simulink model "Test_Board"  (R2020a)
settings: Solver=FixedStepAuto  StartTime=0.0  StopTime=Inf  FixedStep=1e-3  RelTol=1e-3  EnableMultiTasking=on
undefined symbols (not defined in the file): D0, D1, D10, D11, D12, D13, D2, D3, D4, D5, D6, D7, D8, D9, PTA0, PTA1, PTA2, PTB23, PTB9, PTC16, PTC17, PTC2, PTC3, PTC4, PTD0, PTD1, PTD2, PTD3
libraries: frdmk64flib x18, dspstat3 x1
settings Model: ExtModeTrigDuration=5  Creator=Luis  LastModifiedBy=jordanbierbrier
settings OptimizationCC: EnhancedBackFolding=on  PassReuseOutputArgsAs=Individual arguments  ZeroExternalMemoryAtStartup=off  ZeroInternalMemoryAtStartup=off  MaxStackSize=64  OptimizeBlockOrder=speed  DifferentSizesBufferReuse=on  OptimizationCustomize=off  EfficientTunableParamExpr=on
settings DebuggingCC: ParameterTunabilityLossMsg=error
settings HardwareCC: ProdBitPerPointer=32  ProdBitPerSizeT=32  ProdBitPerPtrDiffT=32  ProdLargestAtomicInteger=Long  ProdLargestAtomicFloat=Double  ProdWordSize=32  ProdHWDeviceType=ARM Compatible->ARM Cortex
settings SFSimCC: MATLABDynamicMemAlloc=off
settings RTWCC: SystemTargetFile=ert.tlc  HardwareBoard=NXP FRDM-K64F  TemplateMakefile=ert_default_tmf  Toolchain=GNU Tools for ARM Embedded Processors
settings CodeAppCC: ForceParamTrailComments=on  IgnoreCustomStorageClasses=off  OperatorAnnotations=on  SimulinkDataObjDesc=on  SFDataObjDesc=on  InsertBlockDesc=on

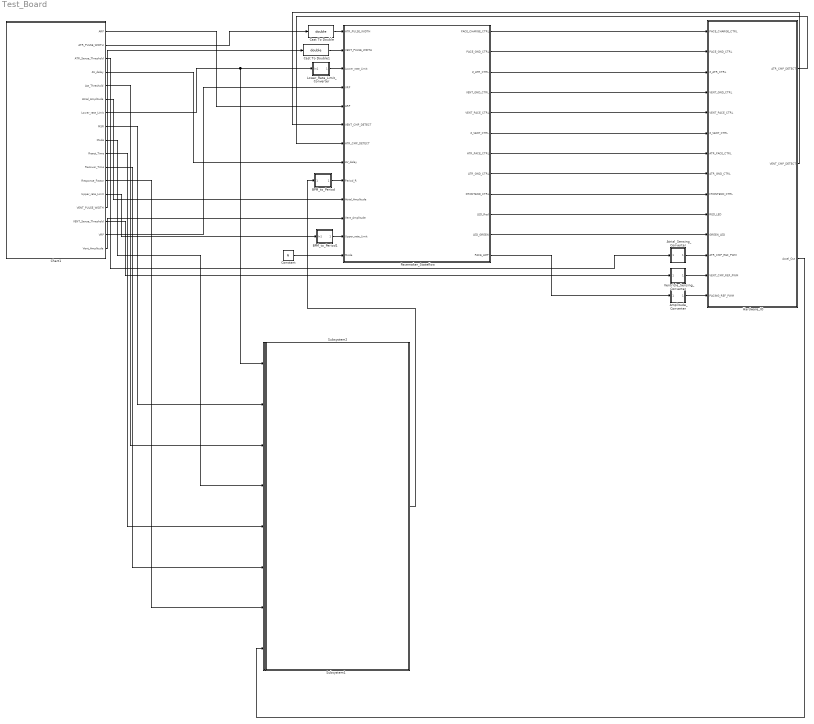
== system Test_Board ==
  Amplitude_Converter : Subsystem
  Atrial_Sensing_Converter : Subsystem
  BPM_to_Period : Subsystem
  BPM_to_Period1 : Subsystem
  Cast To Double : DataTypeConversion  OutDataTypeStr=double
  Cast To Double1 : DataTypeConversion  OutDataTypeStr=double
  Chart1 : Stateflow chart  TreatAsAtomicUnit=on
  Constant : Constant  Value=6  OutDataTypeStr=uint8
  Hardware_IO : Subsystem
  Lower_Rate_Limit_Converter : Subsystem
  "Pacemaker_Stateflow " : Stateflow chart  TreatAsAtomicUnit=on
      settings: PortSchema="{\"entries\":[{\"content\":{\"sides\":[{\"content\":{\"connectorIds\":[\"In1\",\"In4\",\"In2\",\"In5\",\"In6\",\"In7\",\"In8\",\"In9\",\"In10\",\"In11\",\"In12\",\"In13\",\"In3\"]},\"type\":\"ConnectorPlacement.EquallySpacedRectSide\",\"uuid\":\"f97b12ff-cb00-4386-a373-7143c3a8b48d\"},{\"content\":{\"connectorIds\":[\"Out1\",\"Out2\",\"Out3\",\"Out4\",\"Out5\",\"Out6\",\"Out7\",\"Out8\",\"Out9\",\"Out10\",\"Out11\",\"Out12\"],\"side\":\"RIGHT\"},\"type\":\"ConnectorPlacement.EquallySpacedRectSide\",\"uuid\":\"90163773-f9d1-46de-bd72-9589b8539202\"},{\"content\":{\"connectorIds\":[],\"side\":\"TOP\"},\"type\":\"ConnectorPlacement.EquallySpacedRectSide\",\"uuid\":\"f8a54119-a7c4-4071-8260-df405210e670\"},{\"content\":{\"connectorIds\":[],\"side\":\"BOTTOM\"},\"type\":\"ConnectorPlacement.EquallySpacedRectSide\",\"uuid\":\"70f9d800-d0b8-46e1-812e-9f4712f7acbd\"}]},\"type\":\"ConnectorPlacement.EquallySpacedConnector\",\"uuid\":\"47f7c40c-c42b-42f7-beed-99d299c6cdee\"}],\"packageUris\":[\"http://schema.mathworks.com/mf0/Connector/19700101\"],\"version\":\"1.0\"}"
  Subsystem1 : Subsystem
  Subsystem2 : Subsystem
  Ventricle_Sensing_Converter : Subsystem
  wires:
  Amplitude_Converter/1(Out1) -> Hardware_IO/14(PACING_REF_PWM)
  Chart1/13(Upper_rate_Limit) -> BPM_to_Period1/1(In1)
  Chart1/17(Vent_Amplitude) -> "Pacemaker_Stateflow "/12(Vent_Amplitude)
  Lower_Rate_Limit_Converter/1(Out1) -> "Pacemaker_Stateflow "/2(Lower_rate_Limit)
  Chart1/1(ARP) -> "Pacemaker_Stateflow "/6(ARP)
  BPM_to_Period1/1(Out1) -> "Pacemaker_Stateflow "/13(Upper_rate_Limit)
  "Pacemaker_Stateflow "/12(PACE_AMP) -> Amplitude_Converter/1(In1)
  Chart1/6(Atrial_Amplitude) -> "Pacemaker_Stateflow "/11(Atrial_Amplitude)
  Chart1/14(VENT_PULSE_WIDTH) -> Cast To Double1/1
  "Pacemaker_Stateflow "/2(PACE_GND_CTRL) -> Hardware_IO/2(PACE_GND_CTRL)
  "Pacemaker_Stateflow "/9(FRONTEND_CTRL) -> Hardware_IO/9(FRONTEND_CTRL)
  Chart1/10(React_Time) -> Subsystem1/5(Reaction)
  Chart1/12(Response_Factor) -> Subsystem1/7(Response_Factor)
  Cast To Double1/1 -> "Pacemaker_Stateflow "/4(VENT_PULSE_WIDTH)
  Chart1/3(ATR_Sense_Threshold) -> Atrial_Sensing_Converter/1(In1)
  "Pacemaker_Stateflow "/10(LED_Red) -> Hardware_IO/10(RED_LED)
  Chart1/4(AV_delay) -> "Pacemaker_Stateflow "/9(AV_delay)
  "Pacemaker_Stateflow "/7(ATR_PACE_CTRL) -> Hardware_IO/7(ATR_PACE_CTRL)
  "Pacemaker_Stateflow "/3(Z_ATR_CTRL) -> Hardware_IO/3(Z_ATR_CTRL)
  "Pacemaker_Stateflow "/8(ATR_GND_CTRL) -> Hardware_IO/8(ATR_GND_CTRL)
  "Pacemaker_Stateflow "/11(LED_GREEN) -> Hardware_IO/11(GREEN_LED)
  Chart1/2(ATR_PULSE_WIDTH) -> Cast To Double/1
  Chart1/7(Lower_rate_Limit) -> Subsystem1/1(Lower_Rate), Lower_Rate_Limit_Converter/1(In1)
  Ventricle_Sensing_Converter/1(Out1) -> Hardware_IO/13(VENT_CMP_REF_PWM)
  "Pacemaker_Stateflow "/4(VENT_GND_CTRL) -> Hardware_IO/4(VENT_GND_CTRL)
  Chart1/15(VENT_Sense_Threshold) -> Ventricle_Sensing_Converter/1(In1)
  Subsystem1/1(BPM_R) -> BPM_to_Period/1(BPM_R)
  BPM_to_Period/1(Out1) -> "Pacemaker_Stateflow "/10(Period_R)
  "Pacemaker_Stateflow "/1(PACE_CHARGE_CTRL) -> Hardware_IO/1(PACE_CHARGE_CTRL)
  Chart1/8(MSR) -> Subsystem1/2(MSR)
  Chart1/5(Act_Threshold) -> Subsystem1/3(Activity_Thresh)
  Atrial_Sensing_Converter/1(Out1) -> Hardware_IO/12(ATR_CMP_REF_PWM)
  Hardware_IO/2(VENT_CMP_DETECT) -> "Pacemaker_Stateflow "/7(VENT_CMP_DETECT)
  "Pacemaker_Stateflow "/5(VENT_PACE_CTRL) -> Hardware_IO/5(VENT_PACE_CTRL)
  Chart1/9(Mode) -> Subsystem1/4(Mode)
  Chart1/16(VRP) -> "Pacemaker_Stateflow "/5(VRP)
  Hardware_IO/1(ATR_CMP_DETECT) -> "Pacemaker_Stateflow "/8(ATR_CMP_DETECT)
  "Pacemaker_Stateflow "/6(Z_VENT_CTRL) -> Hardware_IO/6(Z_VENT_CTRL)
  Cast To Double/1 -> "Pacemaker_Stateflow "/1(ATR_PULSE_WIDTH)
  Chart1/11(Recover_Time) -> Subsystem1/6(Recovery)
  Hardware_IO/3(Accel_Out) -> Subsystem1/8(Accel_Out)
  Constant/1 -> "Pacemaker_Stateflow "/3(Mode)

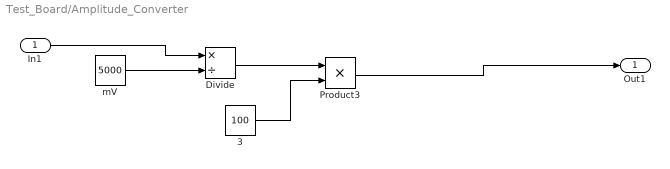
== system Test_Board/Amplitude_Converter ==
  In1 : Inport
  3 : Constant  Value=100  OutDataTypeStr=double
  Divide : Product  Inputs=*/  OutDataTypeStr=double  RndMeth=Nearest
  Product3 : Product  OutDataTypeStr=double
  mV : Constant  Value=5000  OutDataTypeStr=double
  Out1 : Outport
  wires:
  Product3/1 -> Out1/1
  3/1 -> Product3/2
  In1/1 -> Divide/1
  Divide/1 -> Product3/1
  mV/1 -> Divide/2

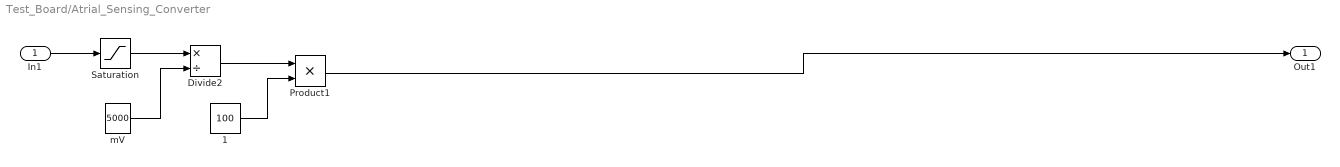
== system Test_Board/Atrial_Sensing_Converter ==
  In1 : Inport
  1 : Constant  Value=100  OutDataTypeStr=uint16
  Divide2 : Product  Inputs=*/  OutDataTypeStr=single
  Product1 : Product  OutDataTypeStr=uint16
  Saturation : Saturate  UpperLimit=4000  LowerLimit=650  LinearizeAsGain=off  OutDataTypeStr=double
  mV : Constant  Value=5000  OutDataTypeStr=double
  Out1 : Outport
  wires:
  Product1/1 -> Out1/1
  1/1 -> Product1/2
  Divide2/1 -> Product1/1
  mV/1 -> Divide2/2
  In1/1 -> Saturation/1
  Saturation/1 -> Divide2/1

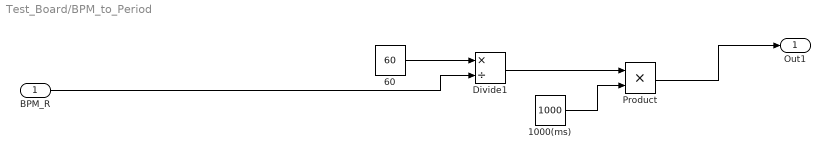
== system Test_Board/BPM_to_Period ==
  BPM_R : Inport
  1000(ms) : Constant  Value=1000  OutDataTypeStr=uint16
  60 : Constant  Value=60  OutDataTypeStr=uint16
  Divide1 : Product  Inputs=*/
  Product : Product  OutDataTypeStr=uint16
  Out1 : Outport
  wires:
  60/1 -> Divide1/1
  BPM_R/1 -> Divide1/2
  Product/1 -> Out1/1
  Divide1/1 -> Product/1
  1000(ms)/1 -> Product/2

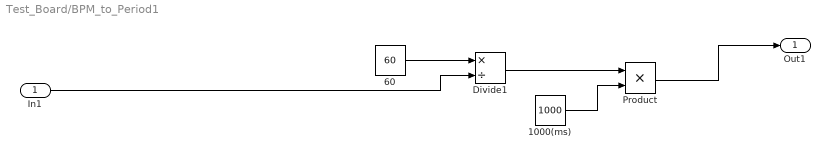
== system Test_Board/BPM_to_Period1 ==
  In1 : Inport
  1000(ms) : Constant  Value=1000  OutDataTypeStr=uint16
  60 : Constant  Value=60  OutDataTypeStr=uint16
  Divide1 : Product  Inputs=*/
  Product : Product  OutDataTypeStr=uint16
  Out1 : Outport
  wires:
  60/1 -> Divide1/1
  In1/1 -> Divide1/2
  Product/1 -> Out1/1
  Divide1/1 -> Product/1
  1000(ms)/1 -> Product/2

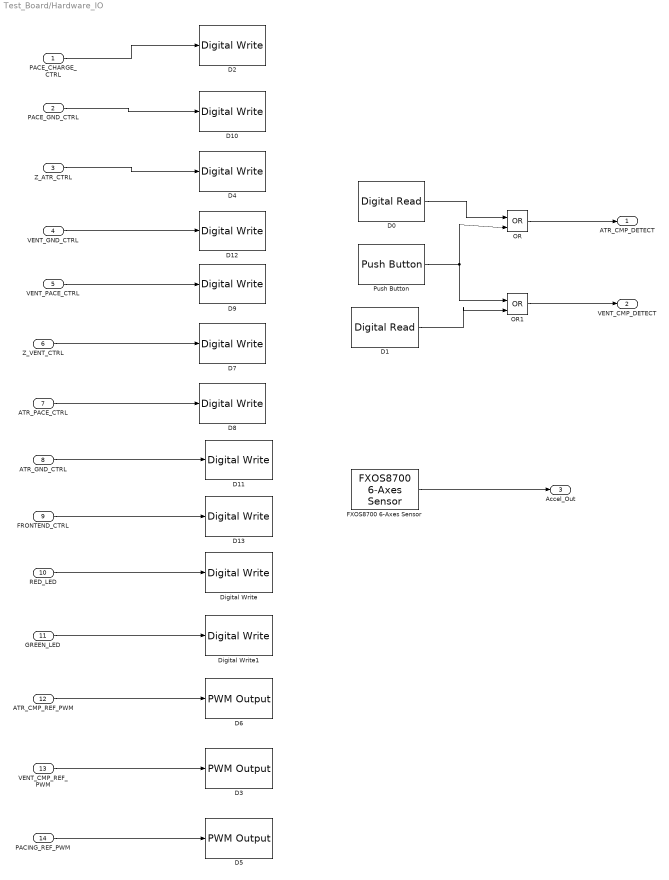
== system Test_Board/Hardware_IO ==
  PACE_CHARGE_CTRL : Inport
  PACE_GND_CTRL : Inport  Port=2
  Z_ATR_CTRL : Inport  Port=3
  VENT_GND_CTRL : Inport  Port=4
  VENT_PACE_CTRL : Inport  Port=5
  Z_VENT_CTRL : Inport  Port=6
  ATR_PACE_CTRL : Inport  Port=7
  ATR_GND_CTRL : Inport  Port=8
  FRONTEND_CTRL : Inport  Port=9
  RED_LED : Inport  Port=10
  GREEN_LED : Inport  Port=11
  ATR_CMP_REF_PWM : Inport  Port=12
  VENT_CMP_REF_PWM : Inport  Port=13
  PACING_REF_PWM : Inport  Port=14
  D0 : frdmk64flib/Digital Read  Whichpin=PTC16 (D0)  SampleTime=-1
  D1 : frdmk64flib/Digital Read  Whichpin=PTC17 (D1)  SampleTime=-1
  D10 : frdmk64flib/Digital Write  Whichpin=PTD0 (D10)
  D11 : frdmk64flib/Digital Write  Whichpin=PTD2 (D11)
  D12 : frdmk64flib/Digital Write  Whichpin=PTD3 (D12)
  D13 : frdmk64flib/Digital Write  Whichpin=PTD1 (D13)
  D2 : frdmk64flib/Digital Write  Whichpin=PTB9 (D2)
  D3 : frdmk64flib/PWM Output  Whichpin=PTA1 (D3)  InitialFrequency=2000  InitialDutyCycle=0
  D4 : frdmk64flib/Digital Write  Whichpin=PTB23 (D4)
  D5 : frdmk64flib/PWM Output  Whichpin=PTA2 (D5)  InitialFrequency=2000  InitialDutyCycle=0
  D6 : frdmk64flib/PWM Output  Whichpin=PTC2 (D6)  InitialFrequency=2000  InitialDutyCycle=0
  D7 : frdmk64flib/Digital Write  Whichpin=PTC3 (D7)
  D8 : frdmk64flib/Digital Write  Whichpin=PTA0 (D8)
  D9 : frdmk64flib/Digital Write  Whichpin=PTC4 (D9)
  Digital Write : frdmk64flib/Digital Write  Whichpin=RED_LED
  Digital Write1 : frdmk64flib/Digital Write  Whichpin=GREEN_LED
  FXOS8700 6-Axes Sensor : frdmk64flib/FXOS8700 6-Axes Sensor  Activesensor=Accelerometer only  ODR=200Hz  HybridODR=400Hz  Accelfullrange=-4g to +4g  SampleTime=0.01
  OR : Logic  Operator=OR  IconShape=distinctive  AllPortsSameDT=off  OutDataTypeStr=boolean
  OR1 : Logic  Operator=OR  IconShape=distinctive  AllPortsSameDT=off  OutDataTypeStr=boolean
  Push Button : frdmk64flib/Push Button  Whichswitch=SW2  SampleTime1=-1
  ATR_CMP_DETECT : Outport
  VENT_CMP_DETECT : Outport  Port=2
  Accel_Out : Outport  Port=3
  wires:
  PACING_REF_PWM/1 -> D5/1
  RED_LED/1 -> Digital Write/1
  Z_ATR_CTRL/1 -> D4/1
  PACE_CHARGE_CTRL/1 -> D2/1
  VENT_GND_CTRL/1 -> D12/1
  D1/1 -> OR1/2
  ATR_PACE_CTRL/1 -> D8/1
  OR1/1 -> VENT_CMP_DETECT/1
  PACE_GND_CTRL/1 -> D10/1
  ATR_GND_CTRL/1 -> D11/1
  OR/1 -> ATR_CMP_DETECT/1
  D0/1 -> OR/1
  ATR_CMP_REF_PWM/1 -> D6/1
  Push Button/1 -> OR1/1, OR/2
  GREEN_LED/1 -> Digital Write1/1
  FRONTEND_CTRL/1 -> D13/1
  VENT_CMP_REF_PWM/1 -> D3/1
  Z_VENT_CTRL/1 -> D7/1
  VENT_PACE_CTRL/1 -> D9/1
  FXOS8700 6-Axes Sensor/1 -> Accel_Out/1

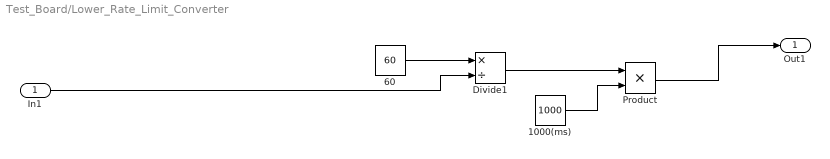
== system Test_Board/Lower_Rate_Limit_Converter ==
  In1 : Inport
  1000(ms) : Constant  Value=1000  OutDataTypeStr=uint16
  60 : Constant  Value=60  OutDataTypeStr=uint16
  Divide1 : Product  Inputs=*/
  Product : Product  OutDataTypeStr=uint16
  Out1 : Outport
  wires:
  60/1 -> Divide1/1
  In1/1 -> Divide1/2
  Product/1 -> Out1/1
  Divide1/1 -> Product/1
  1000(ms)/1 -> Product/2

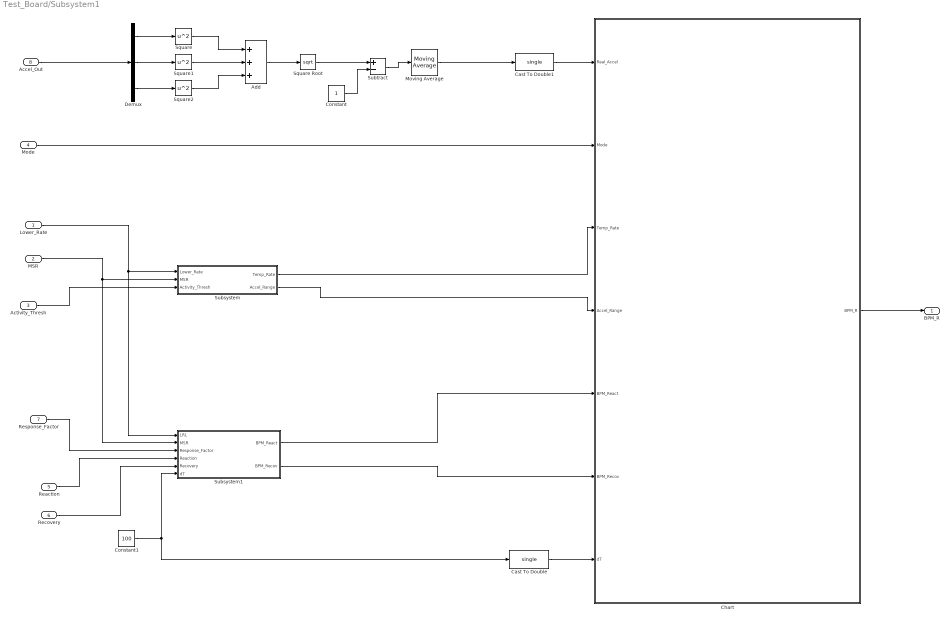
== system Test_Board/Subsystem1 ==
  Lower_Rate : Inport
  MSR : Inport  Port=2
  Activity_Thresh : Inport  Port=3
  Mode : Inport  Port=4
  Reaction : Inport  Port=5
  Recovery : Inport  Port=6
  Response_Factor : Inport  Port=7
  Accel_Out : Inport  Port=8
  Add : Sum  Inputs=+++
  Cast To Double : DataTypeConversion  OutDataTypeStr=single
  Cast To Double1 : DataTypeConversion  OutDataTypeStr=single
  Chart : Stateflow chart  TreatAsAtomicUnit=on
      settings: PortSchema="{\"entries\":[{\"content\":{\"sides\":[{\"content\":{\"connectorIds\":[\"In6\",\"In7\",\"In1\",\"In5\",\"In4\",\"In3\",\"In2\"]},\"type\":\"ConnectorPlacement.EquallySpacedRectSide\",\"uuid\":\"fd37fbd3-e000-4689-ac4c-c5dc5f9ff249\"},{\"content\":{\"connectorIds\":[\"Out1\"],\"side\":\"RIGHT\"},\"type\":\"ConnectorPlacement.EquallySpacedRectSide\",\"uuid\":\"ecd47ea8-5163-45dd-b16f-b562f4f32b7a\"},{\"content\":{\"connectorIds\":[],\"side\":\"TOP\"},\"type\":\"ConnectorPlacement.EquallySpacedRectSide\",\"uuid\":\"5a12f78e-09eb-4424-b8df-032bb9c35282\"}]},\"type\":\"ConnectorPlacement.EquallySpacedConnector\",\"uuid\":\"ee531c1a-9330-4011-aacb-36658e3c3abb\"}],\"packageUris\":[\"http://schema.mathworks.com/mf0/Connector/19700101\"],\"version\":\"1.0\"}"
  Constant : Constant
  Constant1 : Constant  Value=100
  Demux : Demux  Outputs=3
  Moving Average : dspstat3/Moving Average  Method=Sliding window  ForgettingFactorPort=off  SpecifyWindowLength=on  WindowLength=25  ForgettingFactor=0.9  SimulateUsing=Code generation
  Square : Math  Operator=square  SaturateOnIntegerOverflow=on
  Square Root : Sqrt  SaturateOnIntegerOverflow=on
  Square1 : Math  Operator=square  SaturateOnIntegerOverflow=on
  Square2 : Math  Operator=square  SaturateOnIntegerOverflow=on
  Subsystem : Subsystem
  Subsystem1 : Subsystem
  Subtract : Sum  Inputs=+-
  BPM_R : Outport
  wires:
  Demux/3 -> Square2/1
  Subsystem1/1(BPM_React) -> Chart/4(BPM_React)
  Subsystem/1(Temp_Rate) -> Chart/1(Temp_Rate)
  Accel_Out/1 -> Demux/1
  Square/1 -> Add/1
  Demux/2 -> Square1/1
  Mode/1 -> Chart/7(Mode)
  Lower_Rate/1 -> Subsystem/1(Lower_Rate), Subsystem1/1(LRL)
  Response_Factor/1 -> Subsystem1/3(Response_Factor)
  Recovery/1 -> Subsystem1/5(Recovery)
  Add/1 -> Square Root/1
  Subsystem/2(Accel_Range) -> Chart/5(Accel_Range)
  Constant/1 -> Subtract/2
  Subtract/1 -> Moving Average/1
  Square Root/1 -> Subtract/1
  Subsystem1/2(BPM_Recov) -> Chart/3(BPM_Recov)
  Constant1/1 -> Subsystem1/6(dT), Cast To Double/1
  Demux/1 -> Square/1
  Moving Average/1 -> Cast To Double1/1
  Activity_Thresh/1 -> Subsystem/3(Activity_Thresh)
  Square1/1 -> Add/2
  Square2/1 -> Add/3
  Reaction/1 -> Subsystem1/4(Reaction)
  MSR/1 -> Subsystem/2(MSR), Subsystem1/2(MSR)
  Chart/1(BPM_R) -> BPM_R/1
  Cast To Double/1 -> Chart/2(dT)
  Cast To Double1/1 -> Chart/6(Real_Accel)

== system Test_Board/Subsystem2 ==

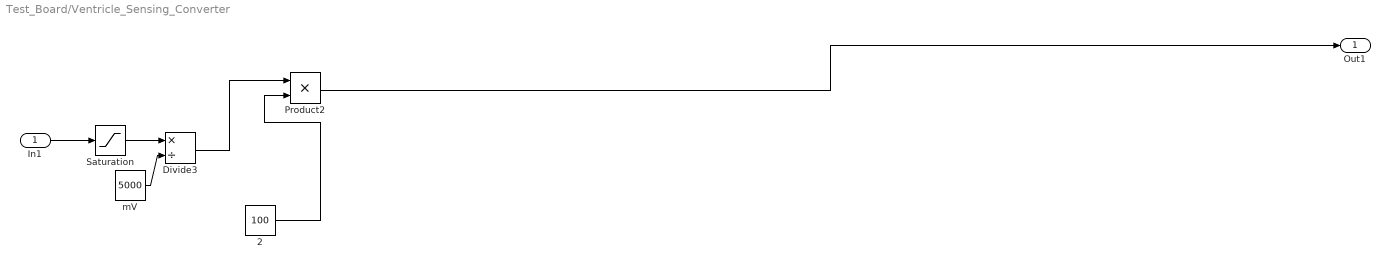
== system Test_Board/Ventricle_Sensing_Converter ==
  In1 : Inport
  2 : Constant  Value=100  OutDataTypeStr=uint16
  Divide3 : Product  Inputs=*/  OutDataTypeStr=single
  Product2 : Product  OutDataTypeStr=uint16
  Saturation : Saturate  UpperLimit=4000  LowerLimit=650  LinearizeAsGain=off  OutDataTypeStr=double
  mV : Constant  Value=5000  OutDataTypeStr=double
  Out1 : Outport
  wires:
  Product2/1 -> Out1/1
  mV/1 -> Divide3/2
  Divide3/1 -> Product2/1
  In1/1 -> Saturation/1
  2/1 -> Product2/2
  Saturation/1 -> Divide3/1

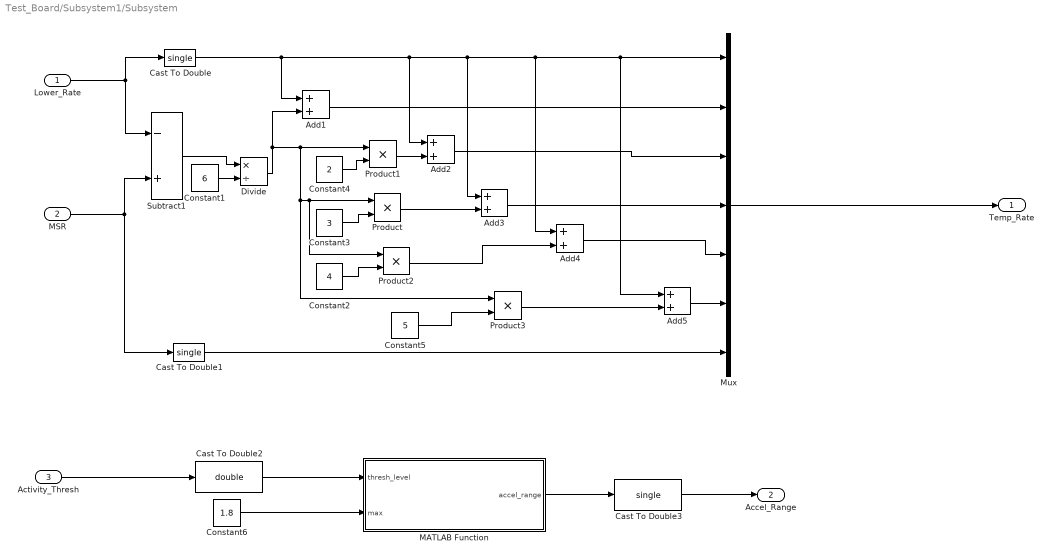
== system Test_Board/Subsystem1/Subsystem ==
  Lower_Rate : Inport
  MSR : Inport  Port=2
  Activity_Thresh : Inport  Port=3
  Add{1,3..5} (4 alike) : Sum  OutDataTypeStr=single
  Add2 : Sum  AccumDataTypeStr=single  OutDataTypeStr=single
  Cast To Double : DataTypeConversion  OutDataTypeStr=single
  Cast To Double1 : DataTypeConversion  OutDataTypeStr=single
  Cast To Double2 : DataTypeConversion  OutDataTypeStr=double
  Cast To Double3 : DataTypeConversion  OutDataTypeStr=single
  Constant1 : Constant  Value=6
  Constant2 : Constant  Value=4
  Constant3 : Constant  Value=3
  Constant4 : Constant  Value=2
  Constant5 : Constant  Value=5
  Constant6 : Constant  Value=1.8  OutDataTypeStr=double
  Divide : Product  Inputs=*/
  MATLAB Function : MATLAB Function  TreatAsAtomicUnit=on
  Mux : Mux  Inputs=7
  Product{,1..3} (4 alike) : Product
  Subtract1 : Sum  Inputs=-+
  Temp_Rate : Outport
  Accel_Range : Outport  Port=2  OutDataTypeStr=single
  wires:
  Constant4/1 -> Product1/2
  Constant1/1 -> Divide/2
  Constant6/1 -> MATLAB Function/2(max)
  Product3/1 -> Add5/2
  MSR/1 -> Cast To Double1/1, Subtract1/2
  Add3/1 -> Mux/4
  Cast To Double/1 -> Add1/1, Mux/1, Add5/1, Add4/1, Add3/1, Add2/1
  Constant3/1 -> Product/2
  Product1/1 -> Add2/2
  Add5/1 -> Mux/6
  Subtract1/1 -> Divide/1
  Activity_Thresh/1 -> Cast To Double2/1
  Divide/1 -> Product3/1, Product2/1, Product/1, Product1/1, Add1/2
  Product2/1 -> Add4/2
  Product/1 -> Add3/2
  Add4/1 -> Mux/5
  Constant2/1 -> Product2/2
  Add2/1 -> Mux/3
  Lower_Rate/1 -> Cast To Double/1, Subtract1/1
  Mux/1 -> Temp_Rate/1
  Cast To Double1/1 -> Mux/7
  Constant5/1 -> Product3/2
  Add1/1 -> Mux/2
  MATLAB Function/1(accel_range) -> Cast To Double3/1
  Cast To Double2/1 -> MATLAB Function/1(thresh_level)
  Cast To Double3/1 -> Accel_Range/1

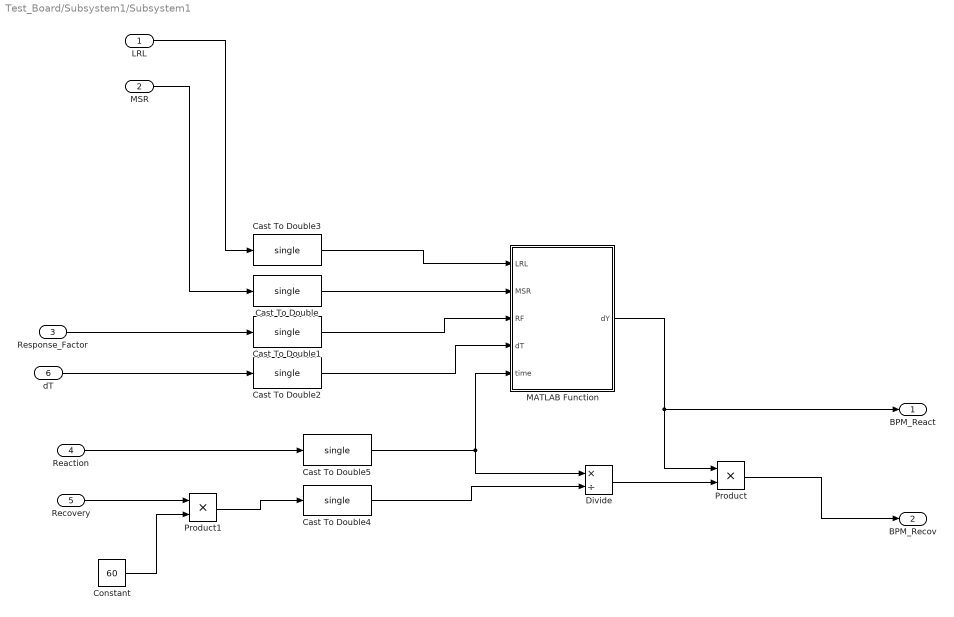
== system Test_Board/Subsystem1/Subsystem1 ==
  LRL : Inport
  MSR : Inport  Port=2
  Response_Factor : Inport  Port=3
  Reaction : Inport  Port=4
  Recovery : Inport  Port=5
  dT : Inport  Port=6
  Cast To Double{,1..5} (6 alike) : DataTypeConversion  OutDataTypeStr=single
  Constant : Constant  Value=60
  Divide : Product  Inputs=*/
  MATLAB Function : MATLAB Function  TreatAsAtomicUnit=on
  Product : Product
  Product1 : Product
  BPM_React : Outport
  BPM_Recov : Outport  Port=2
  wires:
  Product1/1 -> Cast To Double4/1
  Constant/1 -> Product1/2
  Recovery/1 -> Product1/1
  Reaction/1 -> Cast To Double5/1
  Cast To Double5/1 -> MATLAB Function/5(time), Divide/1
  Cast To Double/1 -> MATLAB Function/2(MSR)
  MSR/1 -> Cast To Double/1
  MATLAB Function/1(dY) -> Product/1, BPM_React/1
  Response_Factor/1 -> Cast To Double1/1
  Cast To Double1/1 -> MATLAB Function/3(RF)
  Cast To Double4/1 -> Divide/2
  Cast To Double2/1 -> MATLAB Function/4(dT)
  LRL/1 -> Cast To Double3/1
  Divide/1 -> Product/2
  Cast To Double3/1 -> MATLAB Function/1(LRL)
  dT/1 -> Cast To Double2/1
  Product/1 -> BPM_Recov/1

== stateflow chart Test_Board/Chart1 ==
  settings: executeAtInitialization=1
  state INTIAL
    entry:
    Mode = 6;
    Lower_rate_Limit=50;
    Upper_rate_Limit = 150;
    Atrial_Amplitude=5000;
    Vent_Amplitude=5000;
    ATR_PULSE_WIDTH=1;
    VENT_PULSE_WIDTH=1;
    ATR_Sense_Threshold=2750;
    VENT_Sense_Threshold=2750;
    ARP=250;
    VRP=320;
    AV_delay=100;
    React_Time=10;
    Recover_Time=5;
    Response_Factor=16;
    Act_Threshold=1;
    MSR=120;
  (default) -> INTIAL
  data: ARP output uint16; ATR_PULSE_WIDTH output single; ATR_Sense_Threshold output uint16; AV_delay output uint16; Act_Threshold output uint8; Atrial_Amplitude output uint16; Lower_rate_Limit output uint16; MSR output uint16; Mode output uint8; React_Time output uint16; Recover_Time output uint16; Response_Factor output uint8; Upper_rate_Limit output uint16; VENT_PULSE_WIDTH output single; VENT_Sense_Threshold output uint16; VRP output uint16; Vent_Amplitude output uint16

== stateflow chart Test_Board/Pacemaker_Stateflow  ==
  state AOO
    state AOO_CHARGING
      entry:
      %Charge C22
      ATR_PACE_CTRL=false;
      VENT_PACE_CTRL=false;
      PACE_CHARGE_CTRL=true;
      %Discharge C21
      PACE_GND_CTRL=true;
      Z_VENT_CTRL=false;
      Z_ATR_CTRL=false;
      ATR_GND_CTRL=true;
      PACE_AMP = Atrial_Amplitude;
      VENT_GND_CTRL=false;
      LED_Red = false;
    state AOO_DISCHARGING
      entry:
      %Discharge C22 into ATR
      %Charge C21
      PACE_CHARGE_CTRL=false;
      PACE_GND_CTRL=true;
      ATR_PACE_CTRL=true;
      ATR_GND_CTRL=false;
      Z_VENT_CTRL=false;
      Z_ATR_CTRL=false;
      VENT_GND_CTRL=false;
      VENT_PACE_CTRL=false;
      LED_Red = true;
    AOO_DISCHARGING -> AOO_CHARGING : after(ATR_PULSE_WIDTH,msec)
    AOO_CHARGING -> AOO_DISCHARGING [order 2] : after(Lower_rate_Limit - ATR_PULSE_WIDTH,msec)
  state DOOR [group]
    state DOOR_CHARGING_V
      entry:
      %Charge C22
      VENT_PACE_CTRL=false;
      ATR_PACE_CTRL=false;
      PACE_CHARGE_CTRL=true;
      %Discharge C21 to V
      PACE_GND_CTRL=true;
      Z_VENT_CTRL=false;
      Z_ATR_CTRL=false;
      ATR_PACE_CTRL=false;
      ATR_GND_CTRL=false;
      VENT_GND_CTRL=true;
      LED_GREEN = false;
      %Set PACING_REF_PWM
      PACE_AMP=Atrial_Amplitude;
    state DOOR_PACE_A
      entry:
      %Discharge C22 into ATR
      %Charge C21
      PACE_CHARGE_CTRL=false;
      PACE_GND_CTRL=true;
      ATR_PACE_CTRL=true;
      ATR_GND_CTRL=false;
      Z_VENT_CTRL=false;
      Z_ATR_CTRL=false;
      VENT_GND_CTRL=false;
      VENT_PACE_CTRL=false;
      LED_Red = true;
    state DOOR_CHARGING_A
      entry:
      %Charge C22
      ATR_PACE_CTRL=false;
      VENT_PACE_CTRL=false;
      PACE_CHARGE_CTRL=true;
      %Discharge C21
      PACE_GND_CTRL=true;
      Z_VENT_CTRL=false;
      Z_ATR_CTRL=false;
      ATR_GND_CTRL=true;
      VENT_GND_CTRL=false;
      LED_Red = false;
      %Set PACING_REF_PWM
      PACE_AMP=Vent_Amplitude
    state DOOR_PACE_V
      entry:
      %Discharge C22 into VENT
      %Charge C21
      PACE_CHARGE_CTRL=false;
      PACE_GND_CTRL=true;
      ATR_PACE_CTRL=false;
      ATR_GND_CTRL=false;
      Z_ATR_CTRL=false
      Z_VENT_CTRL=false;
      VENT_GND_CTRL=false;
      VENT_PACE_CTRL=true;
      LED_GREEN = true;
    DOOR_CHARGING_V -> DOOR_PACE_A [order 2] : after(Period_R - (AV_delay+VENT_PULSE_WIDTH),msec)
    DOOR_PACE_A -> DOOR_CHARGING_A : after(ATR_PULSE_WIDTH,msec)
    DOOR_PACE_V -> DOOR_CHARGING_V : after(VENT_PULSE_WIDTH, msec)
    DOOR_CHARGING_A -> DOOR_PACE_V : after(AV_delay - ATR_PULSE_WIDTH,msec)
  state VOO [group]
    state VOO_DISCHARGE
      entry:
      %Discharge C22 into VENT
      %Charge C21
      PACE_CHARGE_CTRL=false;
      PACE_GND_CTRL=true;
      ATR_PACE_CTRL=false;
      ATR_GND_CTRL=false;
      Z_ATR_CTRL=false
      Z_VENT_CTRL=false;
      VENT_GND_CTRL=false;
      VENT_PACE_CTRL=true;
      LED_GREEN = true;
    state VOO_CHARGING
      entry:
      %Charge C22
      VENT_PACE_CTRL=false;
      ATR_PACE_CTRL=false;
      PACE_CHARGE_CTRL=true;
      %Discharge C21
      PACE_GND_CTRL=true;
      Z_VENT_CTRL=false;
      Z_ATR_CTRL=false;
      ATR_PACE_CTRL=false;
      ATR_GND_CTRL=false;
      PACE_AMP = Vent_Amplitude;
      VENT_GND_CTRL=true;
      LED_GREEN = false;
    VOO_DISCHARGE -> VOO_CHARGING : after(VENT_PULSE_WIDTH, msec)
    VOO_CHARGING -> VOO_DISCHARGE [order 2] : after(Lower_rate_Limit - VENT_PULSE_WIDTH, msec)
  state VVIR [group]
    state CHARGING_C22
      entry:
      FRONTEND_CTRL = true;
      PACE_GND_CTRL = true;
      VENT_PACE_CTRL=false;
      ATR_PACE_CTRL=false;
      PACE_CHARGE_CTRL=true;
      Z_VENT_CTRL=false;
      Z_ATR_CTRL=false;
      ATR_GND_CTRL=false;
      PACE_AMP = Vent_Amplitude;
      VENT_GND_CTRL=true;
      LED_GREEN = false;
    state VENTRICAL_PACE
      entry:
      FRONTEND_CTRL = false;
      PACE_GND_CTRL = true;
      VENT_PACE_CTRL=true;
      ATR_PACE_CTRL=false;
      PACE_CHARGE_CTRL=false;
      Z_VENT_CTRL=false;
      Z_ATR_CTRL=false;
      ATR_GND_CTRL=false;
      VENT_GND_CTRL=false;
      LED_GREEN = true;
    state VRP_State
      entry:
      PACE_GND_CTRL = true;
      VENT_PACE_CTRL=false;
      ATR_PACE_CTRL=false;
      PACE_CHARGE_CTRL=true;
      Z_VENT_CTRL=false;
      Z_ATR_CTRL=false;
      ATR_GND_CTRL=false;
      VENT_GND_CTRL=true;
      LED_GREEN = false;
    VVIR.CHARGING_C22 -> VVIR.VENTRICAL_PACE [order 3] : after(Period_R - (VENT_PULSE_WIDTH + VRP), msec)
    VVIR.CHARGING_C22 -> VVIR.VRP_State [order 2] : [VENT_CMP_DETECT == true]
    VVIR.VRP_State -> VVIR.CHARGING_C22 : after(VRP, msec)
    VVIR.VENTRICAL_PACE -> VVIR.VRP_State : after(VENT_PULSE_WIDTH, msec)
  state VVI [group]
    state CHARGING_C22
      entry:
      FRONTEND_CTRL = true;
      PACE_GND_CTRL = true;
      VENT_PACE_CTRL=false;
      ATR_PACE_CTRL=false;
      PACE_CHARGE_CTRL=true;
      Z_VENT_CTRL=false;
      Z_ATR_CTRL=false;
      ATR_GND_CTRL=false;
      PACE_AMP = Vent_Amplitude;
      VENT_GND_CTRL=true;
      LED_GREEN = false;
    state VENTRICAL_PACE
      entry:
      FRONTEND_CTRL = false;
      PACE_GND_CTRL = true;
      VENT_PACE_CTRL=true;
      ATR_PACE_CTRL=false;
      PACE_CHARGE_CTRL=false;
      Z_VENT_CTRL=false;
      Z_ATR_CTRL=false;
      ATR_GND_CTRL=false;
      VENT_GND_CTRL=false;
      LED_GREEN = true;
    state VRP_State
      entry:
      PACE_GND_CTRL = true;
      VENT_PACE_CTRL=false;
      ATR_PACE_CTRL=false;
      PACE_CHARGE_CTRL=true;
      Z_VENT_CTRL=false;
      Z_ATR_CTRL=false;
      ATR_GND_CTRL=false;
      VENT_GND_CTRL=true;
      LED_GREEN = false;
    VVI.CHARGING_C22 -> VVI.VENTRICAL_PACE [order 3] : after((Lower_rate_Limit) - (VENT_PULSE_WIDTH + VRP), msec)
    VVI.CHARGING_C22 -> VVI.VRP_State [order 2] : [VENT_CMP_DETECT == true]
    VVI.VRP_State -> VVI.CHARGING_C22 : after(VRP, msec)
    VVI.VENTRICAL_PACE -> VVI.VRP_State : after(VENT_PULSE_WIDTH, msec)
  state Default
    entry:
    %Charge C22
    ATR_PACE_CTRL=false;
    VENT_PACE_CTRL=false;
    PACE_CHARGE_CTRL=false;
    %Discharge C21
    PACE_GND_CTRL=false;
    Z_VENT_CTRL=false;
    Z_ATR_CTRL=false;
    ATR_GND_CTRL=false;
    VENT_GND_CTRL=false;
    FRONTEND_CTRL=true;
    LED_Red=false;
    LED_GREEN=false;
  state AAIR [group]
    state CHARGING_C22
      entry:
      FRONTEND_CTRL = true;
      PACE_GND_CTRL = true;
      VENT_PACE_CTRL=false;
      ATR_PACE_CTRL=false;
      PACE_CHARGE_CTRL=true;
      Z_VENT_CTRL=false;
      Z_ATR_CTRL=false;
      ATR_GND_CTRL=true;
      PACE_AMP = Atrial_Amplitude;
      VENT_GND_CTRL=false;
      LED_Red = false;
    state ATRIAL_PACE
      entry:
      FRONTEND_CTRL = false;
      PACE_GND_CTRL = true;
      VENT_PACE_CTRL=false;
      ATR_PACE_CTRL=true;
      PACE_CHARGE_CTRL=false;
      Z_VENT_CTRL=false;
      Z_ATR_CTRL=false;
      ATR_GND_CTRL=false;
      VENT_GND_CTRL=false;
      LED_Red = true;
    state ARP_State
      entry:
      PACE_GND_CTRL = true;
      VENT_PACE_CTRL=false;
      ATR_PACE_CTRL=false;
      PACE_CHARGE_CTRL=true;
      Z_VENT_CTRL=false;
      Z_ATR_CTRL=false;
      ATR_GND_CTRL=true;
      VENT_GND_CTRL=false;
      LED_Red = false;
    AAIR.CHARGING_C22 -> AAIR.ATRIAL_PACE [order 3] : after((Period_R) - (ATR_PULSE_WIDTH + ARP), msec)
    AAIR.CHARGING_C22 -> AAIR.ARP_State [order 2] : [ATR_CMP_DETECT == true]
    AAIR.ARP_State -> AAIR.CHARGING_C22 : after(ARP, msec)
    AAIR.ATRIAL_PACE -> AAIR.ARP_State : after(ATR_PULSE_WIDTH, msec)
  state AAI [group]
    state CHARGING_C22
      entry:
      FRONTEND_CTRL = true;
      PACE_GND_CTRL = true;
      VENT_PACE_CTRL=false;
      ATR_PACE_CTRL=false;
      PACE_CHARGE_CTRL=true;
      Z_VENT_CTRL=false;
      Z_ATR_CTRL=false;
      ATR_GND_CTRL=true;
      PACE_AMP = Atrial_Amplitude;
      VENT_GND_CTRL=false;
      LED_Red = false;
    state ATRIAL_PACE
      entry:
      FRONTEND_CTRL = false;
      PACE_GND_CTRL = true;
      VENT_PACE_CTRL=false;
      ATR_PACE_CTRL=true;
      PACE_CHARGE_CTRL=false;
      Z_VENT_CTRL=false;
      Z_ATR_CTRL=false;
      ATR_GND_CTRL=false;
      VENT_GND_CTRL=false;
      LED_Red = true;
    state ARP_State
      entry:
      PACE_GND_CTRL = true;
      VENT_PACE_CTRL=false;
      ATR_PACE_CTRL=false;
      PACE_CHARGE_CTRL=true;
      Z_VENT_CTRL=false;
      Z_ATR_CTRL=false;
      ATR_GND_CTRL=true;
      VENT_GND_CTRL=false;
      LED_Red = false;
    AAI.CHARGING_C22 -> AAI.ATRIAL_PACE [order 3] : after((Lower_rate_Limit) - (ATR_PULSE_WIDTH + ARP), msec)
    AAI.CHARGING_C22 -> AAI.ARP_State [order 2] : [ATR_CMP_DETECT == true]
    AAI.ARP_State -> AAI.CHARGING_C22 : after(ARP, msec)
    AAI.ATRIAL_PACE -> AAI.ARP_State : after(ATR_PULSE_WIDTH, msec)
  state VOOR [group]
    state VOOR_DISCHARGE
      entry:
      %Discharge C22 into VENT
      %Charge C21
      PACE_CHARGE_CTRL=false;
      PACE_GND_CTRL=true;
      ATR_PACE_CTRL=false;
      ATR_GND_CTRL=false;
      Z_ATR_CTRL=false
      Z_VENT_CTRL=false;
      VENT_GND_CTRL=false;
      VENT_PACE_CTRL=true;
      LED_GREEN = true;
    state VOOR_CHARGING
      entry:
      %Charge C22
      VENT_PACE_CTRL=false;
      ATR_PACE_CTRL=false;
      PACE_CHARGE_CTRL=true;
      %Discharge C21
      PACE_GND_CTRL=true;
      Z_VENT_CTRL=false;
      Z_ATR_CTRL=false;
      ATR_PACE_CTRL=false;
      ATR_GND_CTRL=false;
      PACE_AMP = Vent_Amplitude;
      VENT_GND_CTRL=true;
      LED_GREEN = false;
    VOOR_DISCHARGE -> VOOR_CHARGING : after(VENT_PULSE_WIDTH, msec)
    VOOR_CHARGING -> VOOR_DISCHARGE [order 2] : after(Period_R - VENT_PULSE_WIDTH, msec)
  state DOO [group]
    state DOO_CHARGING_V
      entry:
      %Charge C22
      VENT_PACE_CTRL=false;
      ATR_PACE_CTRL=false;
      PACE_CHARGE_CTRL=true;
      %Discharge C21 to V
      PACE_GND_CTRL=true;
      Z_VENT_CTRL=false;
      Z_ATR_CTRL=false;
      ATR_PACE_CTRL=false;
      ATR_GND_CTRL=false;
      VENT_GND_CTRL=true;
      LED_GREEN = false;
      %Set PACING_REF_PWM
      PACE_AMP=Atrial_Amplitude;
    state DOO_PACE_A
      entry:
      %Discharge C22 into ATR
      %Charge C21
      PACE_CHARGE_CTRL=false;
      PACE_GND_CTRL=true;
      ATR_PACE_CTRL=true;
      ATR_GND_CTRL=false;
      Z_VENT_CTRL=false;
      Z_ATR_CTRL=false;
      VENT_GND_CTRL=false;
      VENT_PACE_CTRL=false;
      LED_Red = true;
    state DOO_CHARGING_A
      entry:
      %Charge C22
      ATR_PACE_CTRL=false;
      VENT_PACE_CTRL=false;
      PACE_CHARGE_CTRL=true;
      %Discharge C21
      PACE_GND_CTRL=true;
      Z_VENT_CTRL=false;
      Z_ATR_CTRL=false;
      ATR_GND_CTRL=true;
      VENT_GND_CTRL=false;
      LED_Red = false;
      %Set PACING_REF_PWM
      PACE_AMP=Vent_Amplitude
    state DOO_PACE_V
      entry:
      %Discharge C22 into VENT
      %Charge C21
      PACE_CHARGE_CTRL=false;
      PACE_GND_CTRL=true;
      ATR_PACE_CTRL=false;
      ATR_GND_CTRL=false;
      Z_ATR_CTRL=false
      Z_VENT_CTRL=false;
      VENT_GND_CTRL=false;
      VENT_PACE_CTRL=true;
      LED_GREEN = true;
    DOO_CHARGING_V -> DOO_PACE_A [order 2] : after(Lower_rate_Limit-(AV_delay+VENT_PULSE_WIDTH),msec)
    DOO_PACE_A -> DOO_CHARGING_A : after(ATR_PULSE_WIDTH,msec)
    DOO_PACE_V -> DOO_CHARGING_V : after(VENT_PULSE_WIDTH, msec)
    DOO_CHARGING_A -> DOO_PACE_V : after(AV_delay - ATR_PULSE_WIDTH,msec)
  state AOOR
    state AOOR_DISCHARGING
      entry:
      %Discharge C22 into ATR
      %Charge C21
      PACE_CHARGE_CTRL=false;
      PACE_GND_CTRL=true;
      ATR_PACE_CTRL=true;
      ATR_GND_CTRL=false;
      Z_VENT_CTRL=false;
      Z_ATR_CTRL=false;
      VENT_GND_CTRL=false;
      VENT_PACE_CTRL=false;
      LED_Red = true;
    state AOOR_CHARGING
      entry:
      %Charge C22
      ATR_PACE_CTRL=false;
      VENT_PACE_CTRL=false;
      PACE_CHARGE_CTRL=true;
      %Discharge C21
      PACE_GND_CTRL=true;
      Z_VENT_CTRL=false;
      Z_ATR_CTRL=false;
      ATR_GND_CTRL=true;
      PACE_AMP = Atrial_Amplitude;
      VENT_GND_CTRL=false;
      LED_Red = false;
    AOOR_CHARGING -> AOOR_DISCHARGING [order 2] : after(Period_R - ATR_PULSE_WIDTH,msec)
    AOOR_DISCHARGING -> AOOR_CHARGING : after(ATR_PULSE_WIDTH,msec)
  Default -> DOOR_CHARGING_V [order 8] : [Mode == 10]
  DOOR_CHARGING_V -> Default [order 1] : [Mode~=10]
  Default -> AOO_CHARGING [order 1] : [Mode == 1]
  AOO_CHARGING -> Default [order 1] : [Mode~=1]
  Default -> VOO_CHARGING [order 2] : [Mode == 2]
  VOO_CHARGING -> Default [order 1] : [Mode~=2]
  Default -> VVIR.CHARGING_C22 [order 9] : [Mode ==9]
  VVIR.CHARGING_C22 -> Default [order 1] : [Mode ~= 9]
  Default -> VVI.CHARGING_C22 [order 3] : [Mode == 3]
  VVI.CHARGING_C22 -> Default [order 1] : [Mode ~= 3]
  (default) -> Default
  Default -> Default [order 11] : [Mode == 0 || Lower_rate_Limit>Upper_rate_Limit]
  Default -> AAIR.CHARGING_C22 [order 10] : [Mode == 8]
  AAIR.CHARGING_C22 -> Default [order 1] : [Mode ~= 8]
  Default -> AAI.CHARGING_C22 [order 4] : [Mode == 4]
  AAI.CHARGING_C22 -> Default [order 1] : [Mode ~= 4]
  Default -> VOOR_CHARGING [order 7] : [Mode == 7]
  VOOR_CHARGING -> Default [order 1] : [Mode ~= 7]
  Default -> AOOR_CHARGING [order 6] : [Mode == 6]
  AOOR_CHARGING -> Default [order 1] : [Mode ~=6]
  DOO_CHARGING_V -> Default [order 1] : [Mode ~= 5]
  Default -> DOO_CHARGING_V [order 5] : [Mode == 5]
  data: PACE_CHARGE_CTRL output boolean; PACE_GND_CTRL output boolean; Z_ATR_CTRL output boolean; VENT_GND_CTRL output boolean; VENT_PACE_CTRL output boolean; Z_VENT_CTRL output boolean; ATR_PULSE_WIDTH input double; Lower_rate_Limit input uint16; Mode input uint8; ATR_PACE_CTRL output boolean; ATR_GND_CTRL output boolean; VENT_PULSE_WIDTH input double; VRP input uint16; ARP input uint16; FRONTEND_CTRL output boolean; VENT_CMP_DETECT input boolean; ATR_CMP_DETECT input boolean; LED_Red output boolean; LED_GREEN output boolean; AV_delay input uint16; Period_R input uint16; Atrial_Amplitude input uint16; Vent_Amplitude input uint16; PACE_AMP output uint16; Upper_rate_Limit input uint16

== stateflow chart Test_Board/Subsystem1/Chart ==
  state A
    entry:
    BPM_R = BPM_R + BPM_React;
  state A1
    entry:
    BPM_R = BPM_R + BPM_React;
  state A5
    entry:
    BPM_R = BPM_R + BPM_React;
  state HIGH
    entry:
    if abs (Temp_Rate(6) - BPM_R)  < 1.0
    BPM_R = Temp_Rate(6);
    end
  state S
    entry:
    BPM_R = BPM_R - BPM_Recov
  state MED_H
    entry:
    if abs (Temp_Rate(5) - BPM_R)  < 1.0
    BPM_R = Temp_Rate(5);
    end
  state S1
    entry:
    BPM_R = BPM_R - BPM_Recov;
  state V_HIGH
    entry:
    if abs (Temp_Rate(7) - BPM_R)  < 1.0
    BPM_R = Temp_Rate(7);
    end
  state A2
    entry:
    BPM_R = BPM_R + BPM_React;
  state MED
    entry:
    if abs (Temp_Rate(4) - BPM_R)  < 1.0
    BPM_R = Temp_Rate(4);
    end
  state S2
    entry:
    BPM_R = BPM_R - BPM_Recov;
  state Init
    entry:
    BPM_R = Temp_Rate(1);
  state M_LOW
    entry:
    if abs (Temp_Rate(3) - BPM_R)  < 1.0
    BPM_R = Temp_Rate(3);
    end
  state A3
    entry:
    BPM_R = BPM_R + BPM_React;
  state V_LOW
    entry:
    if abs (Temp_Rate(1) - BPM_R)  < 1.0
    BPM_R = Temp_Rate(1);
    end
  state S3
    entry:
    BPM_R = BPM_R - BPM_Recov;
  state LOW
    entry:
    if abs (Temp_Rate(2) - BPM_R)  < 1.0
    BPM_R = Temp_Rate(2);
    end
  state S5
    entry:
    BPM_R = BPM_R - BPM_Recov;
  state A4
    entry:
    BPM_R = BPM_R + BPM_React;
  state S4
    entry:
    BPM_R = BPM_R - BPM_Recov;
  A -> HIGH
  HIGH -> A [order 3] : [after(dT,msec) && Temp_Rate(6)>BPM_R]
  A1 -> MED_H
  MED_H -> A1 [order 3] : [after(dT,msec) && Temp_Rate(5)>BPM_R]
  V_HIGH -> A5 [order 2] : [after(dT,msec) && Temp_Rate(7)>BPM_R]
  MED_H -> S1 [order 2] : [after(dT,msec) && Temp_Rate(5)<BPM_R]
  HIGH -> S [order 2] : [after(dT,msec) && Temp_Rate(6)<BPM_R]
  S1 -> MED_H
  S -> HIGH
  HIGH -> (junction 30) [order 1] : [Real_Accel<Accel_Range(5) || Real_Accel>Accel_Range(6)]
  (junction 30) -> HIGH [order 2] : [Real_Accel>Accel_Range(5)]
  MED_H -> (junction 30) [order 1] : [Real_Accel<Accel_Range(4) || Real_Accel>Accel_Range(5)]
  (junction 30) -> MED_H [order 3] : [Real_Accel>Accel_Range(4)]
  (junction 30) -> V_HIGH [order 1] : [Real_Accel>Accel_Range(6)]
  V_HIGH -> (junction 30) [order 1] : [Real_Accel<Accel_Range(6)]
  A2 -> MED
  MED -> A2 [order 3] : [after(dT,msec) && Temp_Rate(4)>BPM_R]
  MED -> S2 [order 2] : [after(dT,msec) && Temp_Rate(4)<BPM_R]
  MED -> (junction 30) [order 1] : [Real_Accel<Accel_Range(3) || Real_Accel>Accel_Range(4)]
  S2 -> MED
  (junction 30) -> MED [order 4] : [Real_Accel>Accel_Range(3)]
  (default) -> Init
  Init -> (junction 30) : [Mode >= 6]
  (junction 30) -> Init [order 8] : [Mode <6]
  V_LOW -> (junction 30) [order 1] : [Real_Accel>Accel_Range(1)]
  M_LOW -> (junction 30) [order 1] : [Real_Accel<Accel_Range(2) || Real_Accel>Accel_Range(3)]
  (junction 30) -> M_LOW [order 5] : [Real_Accel>Accel_Range(2)]
  (junction 30) -> V_LOW [order 7] : [Real_Accel>0]
  LOW -> (junction 30) [order 1] : [Real_Accel<Accel_Range(1) || Real_Accel>Accel_Range(2)]
  (junction 30) -> LOW [order 6] : [Real_Accel>Accel_Range(1)]
  A3 -> M_LOW
  M_LOW -> A3 [order 3] : [after(dT,msec) && Temp_Rate(3)>BPM_R]
  M_LOW -> S3 [order 2] : [after(dT,msec) && Temp_Rate(3)<BPM_R]
  S3 -> M_LOW
  V_LOW -> S5 [order 2] : [after(dT,msec) && Temp_Rate(1)<BPM_R]
  S5 -> V_LOW
  A4 -> LOW
  LOW -> A4 [order 3] : [after(dT,msec) && Temp_Rate(2)>BPM_R]
  LOW -> S4 [order 2] : [after(dT,msec) && Temp_Rate(2)<BPM_R]
  S4 -> LOW
  data: Temp_Rate input single; dT input single; BPM_Recov input single; BPM_React input single; Accel_Range input single; Real_Accel input single; BPM_R output single; Mode input uint8

== matlab function Test_Board/Subsystem1/Subsystem/MATLAB Function ==
  data: thresh_level input; accel_range output; max input
function accel_range = fcn(thresh_level, max)
if thresh_level == 2
    AT =0.4;
elseif thresh_level == 3
    AT =0.6 ;
elseif thresh_level == 4
    AT = 0.8;
elseif thresh_level == 5
    AT =1.0 ;
elseif thresh_level == 6
    AT = 1.2;
elseif thresh_level == 7
    AT = 1.4;
else 
    AT = 0.2;
end
AT1 = (max - AT)*(1/6) + AT;
AT2 = (max - AT)*(2/6) + AT;
AT3 = (max - AT)*(3/6) + AT;
AT4 = (max - AT)*(4/6) + AT;
AT5 = (max - AT)*(5/6) + AT;

accel_range = [AT, AT1, AT2, AT3, AT4, AT5];

== matlab function Test_Board/Subsystem1/Subsystem1/MATLAB Function ==
  data: LRL input; MSR input; RF input; dT input; dY output; time input
function dY = fcn(LRL, MSR, RF, dT, time)

dY = ((RF/8)*(MSR-LRL)/(time*1000))*dT;
